simulink model "Project2_Seifi_Ahmadi"  (R2018b)
settings: Solver=ode45  StartTime=0.0  StopTime=900  RelTol=1e-3  EnableMultiTasking=on
values from neighbouring files (symbols this model uses):
  P1 = tf(num,den,'InputDelay',L)    [Project2_Seyfi_Ahmadi.m]
  P2 = tf(num_second,den_second,'InputDelay',190)    [Project2_Seyfi_Ahmadi.m]
undefined symbols (not defined in the file or in its folder): P, tmp
libraries: dspsrcs4 x5
settings Model: TunableVars=tmp  TunableVarsStorageClass=Auto  Creator=Modeer  LastModifiedBy=DearUser
settings DataIOCC: LimitDataPoints=on  SaveFormat=Structure  SaveOutput=off  SaveTime=off
settings OptimizationCC: DefaultParameterBehavior=Inlined  LifeSpan=inf
settings DebuggingCC: UnderspecifiedInitializationDetection=Classic  MergeDetectMultiDrivingBlocksExec=none  SolverPrmCheckMsg=warning  SFUnexpectedBacktrackingDiag=warning  SFNoUnconditionalDefaultTransitionDiag=warning  SFExecutionAtInitializationDiag=none
settings HardwareCC: ProdBitPerPointer=32  ProdBitPerSizeT=32  ProdBitPerPtrDiffT=32  ProdLargestAtomicFloat=None  ProdIntDivRoundTo=Undefined  ProdEndianess=Unspecified  ProdWordSize=32  ProdHWDeviceType=32-bit Generic
settings ModelReferenceCC: PropagateSignalLabelsOutOfModel=off
settings SFSimCC: SimUseLocalCustomCode=off
settings RTWCC: RTWUseLocalCustomCode=off
settings CodeAppCC: StateflowObjectComments=on
settings GRTTargetCC: TargetLangStandard=C89/C90 (ANSI)  GeneratePreprocessorConditionals=Disable all
settings ConfigComp: CovMetricSettings=dw  CovHtmlReporting=on  CovSaveCumulativeToWorkspaceVar=on  CovSaveSingleToWorkspaceVar=on  CovExternalEMLEnable=off

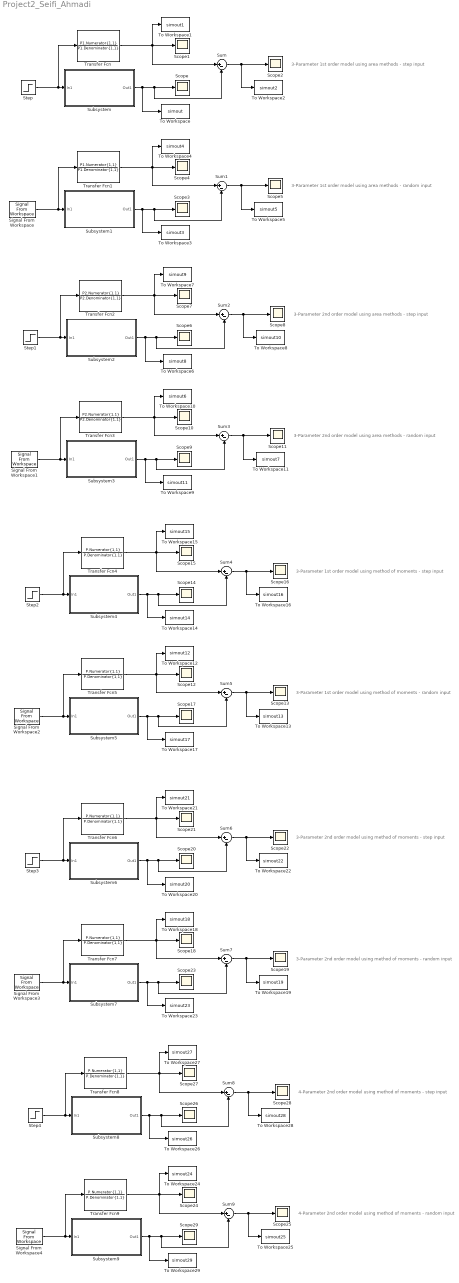
== system Project2_Seifi_Ahmadi ==
  note: 3-Parameter 1st order model using area methods - random input
  note: 3-Parameter 1st order model using area methods - step input
  note: 3-Parameter 2nd order model using area methods - step input
  note: 3-Parameter 2nd order model using area methods - random input
  note: 3-Parameter 1st order model using method of moments - random input
  note: 3-Parameter 1st order model using method of moments - step input
  note: 3-Parameter 2nd order model using method of moments - step input
  note: 3-Parameter 2nd order model using method of moments - random input
  note: 4-Parameter 2nd order model using method of moments - step input
  note: 4-Parameter 2nd order model using method of moments - random input
  Scope{,1..29} (30 alike) : Scope
  Signal From Workspace{,1..4} (5 alike) : dspsrcs4/Signal From Workspace  X=RandomInput  Ts=1  nsamps=1  OutputAfterFinalValue=Setting to zero  ignoreOrWarnInputAndFrameLengths=off  OutputFrames=off
  Step{,1..4} (5 alike) : Step  Time=100  SampleTime=0
  Subsystem : Subsystem  mask{sfcnParam1=tmp}
      mask prompts: sfcnParam1 "tmp:"
      mask help: Simulink:masks:GenSFuncDesc_MD
      mask Help: eval('feval(''rtwprivate'',''rtwhelpview'',''rtw_sfcn_block'')');
  Subsystem1 : Subsystem  mask{sfcnParam1=tmp}
      mask prompts: sfcnParam1 "tmp:"
      mask help: Simulink:masks:GenSFuncDesc_MD
      mask Help: eval('feval(''rtwprivate'',''rtwhelpview'',''rtw_sfcn_block'')');
  Subsystem2 : Subsystem  mask{sfcnParam1=tmp}
      mask prompts: sfcnParam1 "tmp:"
      mask help: Simulink:masks:GenSFuncDesc_MD
      mask Help: eval('feval(''rtwprivate'',''rtwhelpview'',''rtw_sfcn_block'')');
  Subsystem3 : Subsystem  mask{sfcnParam1=tmp}
      mask prompts: sfcnParam1 "tmp:"
      mask help: Simulink:masks:GenSFuncDesc_MD
      mask Help: eval('feval(''rtwprivate'',''rtwhelpview'',''rtw_sfcn_block'')');
  Subsystem4 : Subsystem  mask{sfcnParam1=tmp}
      mask prompts: sfcnParam1 "tmp:"
      mask help: Simulink:masks:GenSFuncDesc_MD
      mask Help: eval('feval(''rtwprivate'',''rtwhelpview'',''rtw_sfcn_block'')');
  Subsystem5 : Subsystem  mask{sfcnParam1=tmp}
      mask prompts: sfcnParam1 "tmp:"
      mask help: Simulink:masks:GenSFuncDesc_MD
      mask Help: eval('feval(''rtwprivate'',''rtwhelpview'',''rtw_sfcn_block'')');
  Subsystem6 : Subsystem  mask{sfcnParam1=tmp}
      mask prompts: sfcnParam1 "tmp:"
      mask help: Simulink:masks:GenSFuncDesc_MD
      mask Help: eval('feval(''rtwprivate'',''rtwhelpview'',''rtw_sfcn_block'')');
  Subsystem7 : Subsystem  mask{sfcnParam1=tmp}
      mask prompts: sfcnParam1 "tmp:"
      mask help: Simulink:masks:GenSFuncDesc_MD
      mask Help: eval('feval(''rtwprivate'',''rtwhelpview'',''rtw_sfcn_block'')');
  Subsystem8 : Subsystem  mask{sfcnParam1=tmp}
      mask prompts: sfcnParam1 "tmp:"
      mask help: Simulink:masks:GenSFuncDesc_MD
      mask Help: eval('feval(''rtwprivate'',''rtwhelpview'',''rtw_sfcn_block'')');
  Subsystem9 : Subsystem  mask{sfcnParam1=tmp}
      mask prompts: sfcnParam1 "tmp:"
      mask help: Simulink:masks:GenSFuncDesc_MD
      mask Help: eval('feval(''rtwprivate'',''rtwhelpview'',''rtw_sfcn_block'')');
  Sum{,1..9} (10 alike) : Sum  Inputs=|+-
  To Workspace : ToWorkspace  VariableName=simout  SaveFormat=Timeseries  SampleTime=-1
  To Workspace1 : ToWorkspace  VariableName=simout1  SaveFormat=Timeseries  SampleTime=-1
  To Workspace10 : ToWorkspace  VariableName=simout6  SaveFormat=Timeseries  SampleTime=-1
  To Workspace11 : ToWorkspace  VariableName=simout7  SaveFormat=Timeseries  SampleTime=-1
  To Workspace12 : ToWorkspace  VariableName=simout12  SaveFormat=Timeseries  SampleTime=-1
  To Workspace13 : ToWorkspace  VariableName=simout13  SaveFormat=Timeseries  SampleTime=-1
  To Workspace14 : ToWorkspace  VariableName=simout14  SaveFormat=Timeseries  SampleTime=-1
  To Workspace15 : ToWorkspace  VariableName=simout15  SaveFormat=Timeseries  SampleTime=-1
  To Workspace16 : ToWorkspace  VariableName=simout16  SaveFormat=Timeseries  SampleTime=-1
  To Workspace17 : ToWorkspace  VariableName=simout17  SaveFormat=Timeseries  SampleTime=-1
  To Workspace18 : ToWorkspace  VariableName=simout18  SaveFormat=Timeseries  SampleTime=-1
  To Workspace19 : ToWorkspace  VariableName=simout19  SaveFormat=Timeseries  SampleTime=-1
  To Workspace2 : ToWorkspace  VariableName=simout2  SaveFormat=Timeseries  SampleTime=-1
  To Workspace20 : ToWorkspace  VariableName=simout20  SaveFormat=Timeseries  SampleTime=-1
  To Workspace21 : ToWorkspace  VariableName=simout21  SaveFormat=Timeseries  SampleTime=-1
  To Workspace22 : ToWorkspace  VariableName=simout22  SaveFormat=Timeseries  SampleTime=-1
  To Workspace23 : ToWorkspace  VariableName=simout23  SaveFormat=Timeseries  SampleTime=-1
  To Workspace24 : ToWorkspace  VariableName=simout24  SaveFormat=Timeseries  SampleTime=-1
  To Workspace25 : ToWorkspace  VariableName=simout25  SaveFormat=Timeseries  SampleTime=-1
  To Workspace26 : ToWorkspace  VariableName=simout26  SaveFormat=Timeseries  SampleTime=-1
  To Workspace27 : ToWorkspace  VariableName=simout27  SaveFormat=Timeseries  SampleTime=-1
  To Workspace28 : ToWorkspace  VariableName=simout28  SaveFormat=Timeseries  SampleTime=-1
  To Workspace29 : ToWorkspace  VariableName=simout29  SaveFormat=Timeseries  SampleTime=-1
  To Workspace3 : ToWorkspace  VariableName=simout3  SaveFormat=Timeseries  SampleTime=-1
  To Workspace4 : ToWorkspace  VariableName=simout4  SaveFormat=Timeseries  SampleTime=-1
  To Workspace5 : ToWorkspace  VariableName=simout5  SaveFormat=Timeseries  SampleTime=-1
  To Workspace6 : ToWorkspace  VariableName=simout8  SaveFormat=Timeseries  SampleTime=-1
  To Workspace7 : ToWorkspace  VariableName=simout9  SaveFormat=Timeseries  SampleTime=-1
  To Workspace8 : ToWorkspace  VariableName=simout10  SaveFormat=Timeseries  SampleTime=-1
  To Workspace9 : ToWorkspace  VariableName=simout11  SaveFormat=Timeseries  SampleTime=-1
  Transfer Fcn : TransferFcn  Numerator=P1.Numerator{1,1}  Denominator=P1.Denominator{1,1}
  Transfer Fcn1 : TransferFcn  Numerator=P1.Numerator{1,1}  Denominator=P1.Denominator{1,1}
  Transfer Fcn2 : TransferFcn  Numerator=P2.Numerator{1,1}  Denominator=P2.Denominator{1,1}
  Transfer Fcn3 : TransferFcn  Numerator=P2.Numerator{1,1}  Denominator=P2.Denominator{1,1}
  Transfer Fcn{4..9} (6 alike) : TransferFcn  Numerator=P.Numerator{1,1}  Denominator=P.Denominator{1,1}
  wires:
  Step/1 -> Transfer Fcn/1, Subsystem/1(In1)
  Subsystem/1(Out1) -> To Workspace/1, Sum/2, Scope/1
  Transfer Fcn/1 -> To Workspace1/1, Scope1/1, Sum/1
  Sum/1 -> To Workspace2/1, Scope2/1
  Subsystem1/1(Out1) -> To Workspace3/1, Sum1/2, Scope3/1
  Signal From Workspace/1 -> Transfer Fcn1/1, Subsystem1/1(In1)
  Transfer Fcn1/1 -> To Workspace4/1, Scope4/1, Sum1/1
  Sum1/1 -> To Workspace5/1, Scope5/1
  Sum3/1 -> To Workspace11/1, Scope11/1
  Transfer Fcn3/1 -> To Workspace10/1, Scope10/1, Sum3/1
  Subsystem2/1(Out1) -> To Workspace6/1, Sum2/2, Scope6/1
  Step1/1 -> Transfer Fcn2/1, Subsystem2/1(In1)
  Transfer Fcn2/1 -> To Workspace7/1, Scope7/1, Sum2/1
  Signal From Workspace1/1 -> Transfer Fcn3/1, Subsystem3/1(In1)
  Subsystem3/1(Out1) -> To Workspace9/1, Sum3/2, Scope9/1
  Sum2/1 -> To Workspace8/1, Scope8/1
  Sum4/1 -> To Workspace16/1, Scope16/1
  Subsystem5/1(Out1) -> To Workspace17/1, Sum5/2, Scope17/1
  Signal From Workspace2/1 -> Transfer Fcn5/1, Subsystem5/1(In1)
  Transfer Fcn4/1 -> To Workspace15/1, Scope15/1, Sum4/1
  Step2/1 -> Transfer Fcn4/1, Subsystem4/1(In1)
  Subsystem4/1(Out1) -> To Workspace14/1, Sum4/2, Scope14/1
  Transfer Fcn5/1 -> To Workspace12/1, Scope12/1, Sum5/1
  Sum5/1 -> To Workspace13/1, Scope13/1
  Subsystem6/1(Out1) -> To Workspace20/1, Sum6/2, Scope20/1
  Transfer Fcn7/1 -> To Workspace18/1, Scope18/1, Sum7/1
  Transfer Fcn6/1 -> To Workspace21/1, Scope21/1, Sum6/1
  Signal From Workspace3/1 -> Transfer Fcn7/1, Subsystem7/1(In1)
  Step3/1 -> Transfer Fcn6/1, Subsystem6/1(In1)
  Sum7/1 -> To Workspace19/1, Scope19/1
  Subsystem7/1(Out1) -> To Workspace23/1, Sum7/2, Scope23/1
  Sum6/1 -> To Workspace22/1, Scope22/1
  Step4/1 -> Transfer Fcn8/1, Subsystem8/1(In1)
  Sum9/1 -> To Workspace25/1, Scope25/1
  Signal From Workspace4/1 -> Transfer Fcn9/1, Subsystem9/1(In1)
  Transfer Fcn8/1 -> To Workspace27/1, Scope27/1, Sum8/1
  Transfer Fcn9/1 -> To Workspace24/1, Scope24/1, Sum9/1
  Sum8/1 -> To Workspace28/1, Scope28/1
  Subsystem8/1(Out1) -> To Workspace26/1, Sum8/2, Scope26/1
  Subsystem9/1(Out1) -> To Workspace29/1, Sum9/2, Scope29/1

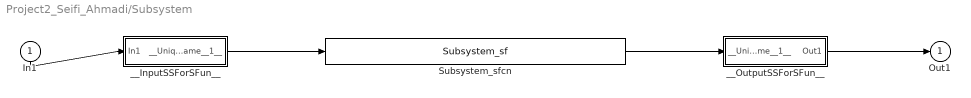
== system Project2_Seifi_Ahmadi/Subsystem ==
  In1 : Inport
  Subsystem_sfcn : S-Function  FunctionName=Subsystem_sf  Parameters=sfcnParam1  SFunctionModules=""  SFunctionDeploymentMode=off  EnableBusSupport=off  mask{rtw_sf_name=Subsystem_sf, showVar=off, sfcnParam1=sfcnParam1}
      mask prompts: rtw_sf_name "Simulink:masks:GenSFuncName_MP"; showVar "Simulink:masks:GenSFuncShowModuleList_MP"; sfcnParam1 "tmp:"
      mask help: Simulink:masks:GenSFuncDesc_MD
      mask init:
      | displist = '';
      | if ~strcmp(get_param(gcb, 'FunctionName'), rtw_sf_name);
      |   set_param(gcb, 'FunctionName', rtw_sf_name);
      | end
      | % Check if we are generating code
      | rtw_mode = false;
      | if strcmpi(get_param(bdroot(gcb),'SimulationStatus'),'Initializing')
      | 	rtw_mode = strcmpi(get_param(bdroot(gcb),'BuildingRTWCode'),'on') && ...
      | 		~strcmpi(get_param(bdroot(gcb),'TargetStyle'),'SimulationTarget');
      | end
      | if showVar || rtw_mode
      | 	if exist('rtwsfunc') == 2 | exist('rtwsfunc') == 6
      | 		tmplist = rtwsfunc(rtw_sf_name,gcb);
      | 		tmplist = DAStudio.message('Simulink:masks:GenSFuncListOfModules_IC', tmplist);
      | 	elseif showVar
      | 		tmplist1 = DAStudio.message('Simulink:masks:GenSFuncListOfModules_IC', '');
      |         tmplist2 = DAStudio.message('Simulink:masks:GenSFuncNotLicensed_IC');
      |         tmplist = [tmplist1 tmplist2];
      |  	end
      | end
      | if showVar
      |   displist = tmplist;
      | end
      settings: CopyFcn=|
      | if ~strcmp(get_param(gcb,'Linkstatus'),'none') && ...
      | ~strcmp(get_param(gcb,'Linkstatus'),'implicit')
      |   set_param(gcb,'LinkStatus','none');
      | end
      mask Help: eval('feval(''rtwprivate'',''rtwhelpview'',''rtw_sfcn_block'')');
      mask Display:
      | port_label('input',1,'In1');
      | port_label('output',1,'Out1');
  __InputSSForSFun__ : Subsystem
  __OutputSSForSFun__ : Subsystem
  Out1 : Outport
  wires:
  In1/1 -> __InputSSForSFun__/1(In1)
  __InputSSForSFun__/1(__UniqueOutportName__1__) -> Subsystem_sfcn/1
  Subsystem_sfcn/1 -> __OutputSSForSFun__/1(__UniqueInportName__1__)
  __OutputSSForSFun__/1(Out1) -> Out1/1

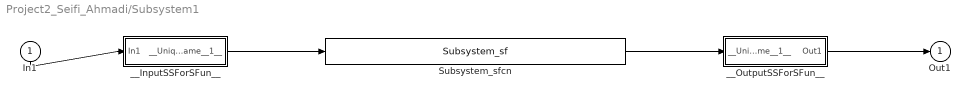
== system Project2_Seifi_Ahmadi/Subsystem1 ==
  In1 : Inport
  Subsystem_sfcn : S-Function  FunctionName=Subsystem_sf  Parameters=sfcnParam1  SFunctionModules=""  SFunctionDeploymentMode=off  EnableBusSupport=off  mask{rtw_sf_name=Subsystem_sf, showVar=off, sfcnParam1=sfcnParam1}
      mask prompts: rtw_sf_name "Simulink:masks:GenSFuncName_MP"; showVar "Simulink:masks:GenSFuncShowModuleList_MP"; sfcnParam1 "tmp:"
      mask help: Simulink:masks:GenSFuncDesc_MD
      mask init: same as Project2_Seifi_Ahmadi/Subsystem/Subsystem_sfcn
      settings: CopyFcn=|
      | if ~strcmp(get_param(gcb,'Linkstatus'),'none') && ...
      | ~strcmp(get_param(gcb,'Linkstatus'),'implicit')
      |   set_param(gcb,'LinkStatus','none');
      | end
      mask Help: eval('feval(''rtwprivate'',''rtwhelpview'',''rtw_sfcn_block'')');
      mask Display:
      | port_label('input',1,'In1');
      | port_label('output',1,'Out1');
  __InputSSForSFun__ : Subsystem
  __OutputSSForSFun__ : Subsystem
  Out1 : Outport
  wires:
  In1/1 -> __InputSSForSFun__/1(In1)
  __InputSSForSFun__/1(__UniqueOutportName__1__) -> Subsystem_sfcn/1
  Subsystem_sfcn/1 -> __OutputSSForSFun__/1(__UniqueInportName__1__)
  __OutputSSForSFun__/1(Out1) -> Out1/1

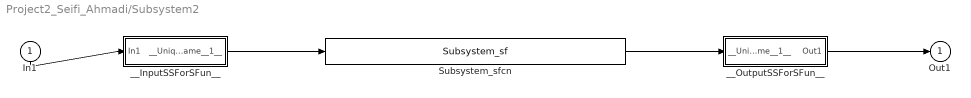
== system Project2_Seifi_Ahmadi/Subsystem2 ==
  In1 : Inport
  Subsystem_sfcn : S-Function  FunctionName=Subsystem_sf  Parameters=sfcnParam1  SFunctionModules=""  SFunctionDeploymentMode=off  EnableBusSupport=off  mask{rtw_sf_name=Subsystem_sf, showVar=off, sfcnParam1=sfcnParam1}
      mask prompts: rtw_sf_name "Simulink:masks:GenSFuncName_MP"; showVar "Simulink:masks:GenSFuncShowModuleList_MP"; sfcnParam1 "tmp:"
      mask help: Simulink:masks:GenSFuncDesc_MD
      mask init: same as Project2_Seifi_Ahmadi/Subsystem/Subsystem_sfcn
      settings: CopyFcn=|
      | if ~strcmp(get_param(gcb,'Linkstatus'),'none') && ...
      | ~strcmp(get_param(gcb,'Linkstatus'),'implicit')
      |   set_param(gcb,'LinkStatus','none');
      | end
      mask Help: eval('feval(''rtwprivate'',''rtwhelpview'',''rtw_sfcn_block'')');
      mask Display:
      | port_label('input',1,'In1');
      | port_label('output',1,'Out1');
  __InputSSForSFun__ : Subsystem
  __OutputSSForSFun__ : Subsystem
  Out1 : Outport
  wires:
  In1/1 -> __InputSSForSFun__/1(In1)
  __InputSSForSFun__/1(__UniqueOutportName__1__) -> Subsystem_sfcn/1
  Subsystem_sfcn/1 -> __OutputSSForSFun__/1(__UniqueInportName__1__)
  __OutputSSForSFun__/1(Out1) -> Out1/1

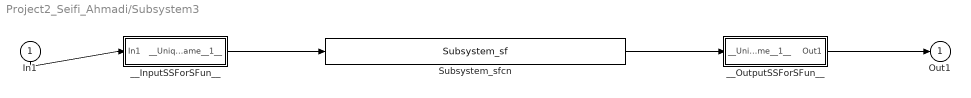
== system Project2_Seifi_Ahmadi/Subsystem3 ==
  In1 : Inport
  Subsystem_sfcn : S-Function  FunctionName=Subsystem_sf  Parameters=sfcnParam1  SFunctionModules=""  SFunctionDeploymentMode=off  EnableBusSupport=off  mask{rtw_sf_name=Subsystem_sf, showVar=off, sfcnParam1=sfcnParam1}
      mask prompts: rtw_sf_name "Simulink:masks:GenSFuncName_MP"; showVar "Simulink:masks:GenSFuncShowModuleList_MP"; sfcnParam1 "tmp:"
      mask help: Simulink:masks:GenSFuncDesc_MD
      mask init: same as Project2_Seifi_Ahmadi/Subsystem/Subsystem_sfcn
      settings: CopyFcn=|
      | if ~strcmp(get_param(gcb,'Linkstatus'),'none') && ...
      | ~strcmp(get_param(gcb,'Linkstatus'),'implicit')
      |   set_param(gcb,'LinkStatus','none');
      | end
      mask Help: eval('feval(''rtwprivate'',''rtwhelpview'',''rtw_sfcn_block'')');
      mask Display:
      | port_label('input',1,'In1');
      | port_label('output',1,'Out1');
  __InputSSForSFun__ : Subsystem
  __OutputSSForSFun__ : Subsystem
  Out1 : Outport
  wires:
  In1/1 -> __InputSSForSFun__/1(In1)
  __InputSSForSFun__/1(__UniqueOutportName__1__) -> Subsystem_sfcn/1
  Subsystem_sfcn/1 -> __OutputSSForSFun__/1(__UniqueInportName__1__)
  __OutputSSForSFun__/1(Out1) -> Out1/1

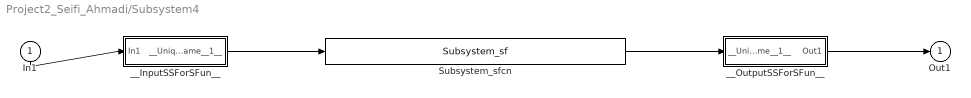
== system Project2_Seifi_Ahmadi/Subsystem4 ==
  In1 : Inport
  Subsystem_sfcn : S-Function  FunctionName=Subsystem_sf  Parameters=sfcnParam1  SFunctionModules=""  SFunctionDeploymentMode=off  EnableBusSupport=off  mask{rtw_sf_name=Subsystem_sf, showVar=off, sfcnParam1=sfcnParam1}
      mask prompts: rtw_sf_name "Simulink:masks:GenSFuncName_MP"; showVar "Simulink:masks:GenSFuncShowModuleList_MP"; sfcnParam1 "tmp:"
      mask help: Simulink:masks:GenSFuncDesc_MD
      mask init: same as Project2_Seifi_Ahmadi/Subsystem/Subsystem_sfcn
      settings: CopyFcn=|
      | if ~strcmp(get_param(gcb,'Linkstatus'),'none') && ...
      | ~strcmp(get_param(gcb,'Linkstatus'),'implicit')
      |   set_param(gcb,'LinkStatus','none');
      | end
      mask Help: eval('feval(''rtwprivate'',''rtwhelpview'',''rtw_sfcn_block'')');
      mask Display:
      | port_label('input',1,'In1');
      | port_label('output',1,'Out1');
  __InputSSForSFun__ : Subsystem
  __OutputSSForSFun__ : Subsystem
  Out1 : Outport
  wires:
  In1/1 -> __InputSSForSFun__/1(In1)
  __InputSSForSFun__/1(__UniqueOutportName__1__) -> Subsystem_sfcn/1
  Subsystem_sfcn/1 -> __OutputSSForSFun__/1(__UniqueInportName__1__)
  __OutputSSForSFun__/1(Out1) -> Out1/1

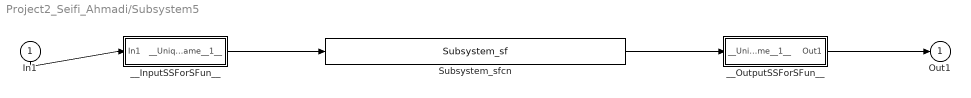
== system Project2_Seifi_Ahmadi/Subsystem5 ==
  In1 : Inport
  Subsystem_sfcn : S-Function  FunctionName=Subsystem_sf  Parameters=sfcnParam1  SFunctionModules=""  SFunctionDeploymentMode=off  EnableBusSupport=off  mask{rtw_sf_name=Subsystem_sf, showVar=off, sfcnParam1=sfcnParam1}
      mask prompts: rtw_sf_name "Simulink:masks:GenSFuncName_MP"; showVar "Simulink:masks:GenSFuncShowModuleList_MP"; sfcnParam1 "tmp:"
      mask help: Simulink:masks:GenSFuncDesc_MD
      mask init: same as Project2_Seifi_Ahmadi/Subsystem/Subsystem_sfcn
      settings: CopyFcn=|
      | if ~strcmp(get_param(gcb,'Linkstatus'),'none') && ...
      | ~strcmp(get_param(gcb,'Linkstatus'),'implicit')
      |   set_param(gcb,'LinkStatus','none');
      | end
      mask Help: eval('feval(''rtwprivate'',''rtwhelpview'',''rtw_sfcn_block'')');
      mask Display:
      | port_label('input',1,'In1');
      | port_label('output',1,'Out1');
  __InputSSForSFun__ : Subsystem
  __OutputSSForSFun__ : Subsystem
  Out1 : Outport
  wires:
  In1/1 -> __InputSSForSFun__/1(In1)
  __InputSSForSFun__/1(__UniqueOutportName__1__) -> Subsystem_sfcn/1
  Subsystem_sfcn/1 -> __OutputSSForSFun__/1(__UniqueInportName__1__)
  __OutputSSForSFun__/1(Out1) -> Out1/1

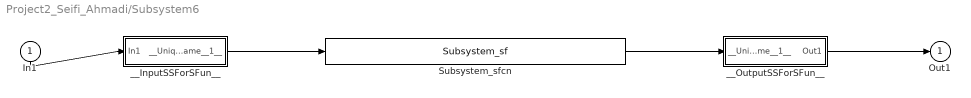
== system Project2_Seifi_Ahmadi/Subsystem6 ==
  In1 : Inport
  Subsystem_sfcn : S-Function  FunctionName=Subsystem_sf  Parameters=sfcnParam1  SFunctionModules=""  SFunctionDeploymentMode=off  EnableBusSupport=off  mask{rtw_sf_name=Subsystem_sf, showVar=off, sfcnParam1=sfcnParam1}
      mask prompts: rtw_sf_name "Simulink:masks:GenSFuncName_MP"; showVar "Simulink:masks:GenSFuncShowModuleList_MP"; sfcnParam1 "tmp:"
      mask help: Simulink:masks:GenSFuncDesc_MD
      mask init: same as Project2_Seifi_Ahmadi/Subsystem/Subsystem_sfcn
      settings: CopyFcn=|
      | if ~strcmp(get_param(gcb,'Linkstatus'),'none') && ...
      | ~strcmp(get_param(gcb,'Linkstatus'),'implicit')
      |   set_param(gcb,'LinkStatus','none');
      | end
      mask Help: eval('feval(''rtwprivate'',''rtwhelpview'',''rtw_sfcn_block'')');
      mask Display:
      | port_label('input',1,'In1');
      | port_label('output',1,'Out1');
  __InputSSForSFun__ : Subsystem
  __OutputSSForSFun__ : Subsystem
  Out1 : Outport
  wires:
  In1/1 -> __InputSSForSFun__/1(In1)
  __InputSSForSFun__/1(__UniqueOutportName__1__) -> Subsystem_sfcn/1
  Subsystem_sfcn/1 -> __OutputSSForSFun__/1(__UniqueInportName__1__)
  __OutputSSForSFun__/1(Out1) -> Out1/1

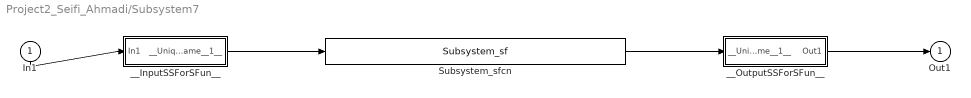
== system Project2_Seifi_Ahmadi/Subsystem7 ==
  In1 : Inport
  Subsystem_sfcn : S-Function  FunctionName=Subsystem_sf  Parameters=sfcnParam1  SFunctionModules=""  SFunctionDeploymentMode=off  EnableBusSupport=off  mask{rtw_sf_name=Subsystem_sf, showVar=off, sfcnParam1=sfcnParam1}
      mask prompts: rtw_sf_name "Simulink:masks:GenSFuncName_MP"; showVar "Simulink:masks:GenSFuncShowModuleList_MP"; sfcnParam1 "tmp:"
      mask help: Simulink:masks:GenSFuncDesc_MD
      mask init: same as Project2_Seifi_Ahmadi/Subsystem/Subsystem_sfcn
      settings: CopyFcn=|
      | if ~strcmp(get_param(gcb,'Linkstatus'),'none') && ...
      | ~strcmp(get_param(gcb,'Linkstatus'),'implicit')
      |   set_param(gcb,'LinkStatus','none');
      | end
      mask Help: eval('feval(''rtwprivate'',''rtwhelpview'',''rtw_sfcn_block'')');
      mask Display:
      | port_label('input',1,'In1');
      | port_label('output',1,'Out1');
  __InputSSForSFun__ : Subsystem
  __OutputSSForSFun__ : Subsystem
  Out1 : Outport
  wires:
  In1/1 -> __InputSSForSFun__/1(In1)
  __InputSSForSFun__/1(__UniqueOutportName__1__) -> Subsystem_sfcn/1
  Subsystem_sfcn/1 -> __OutputSSForSFun__/1(__UniqueInportName__1__)
  __OutputSSForSFun__/1(Out1) -> Out1/1

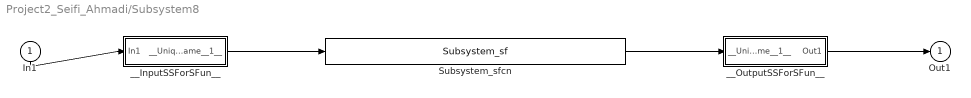
== system Project2_Seifi_Ahmadi/Subsystem8 ==
  In1 : Inport
  Subsystem_sfcn : S-Function  FunctionName=Subsystem_sf  Parameters=sfcnParam1  SFunctionModules=""  SFunctionDeploymentMode=off  EnableBusSupport=off  mask{rtw_sf_name=Subsystem_sf, showVar=off, sfcnParam1=sfcnParam1}
      mask prompts: rtw_sf_name "Simulink:masks:GenSFuncName_MP"; showVar "Simulink:masks:GenSFuncShowModuleList_MP"; sfcnParam1 "tmp:"
      mask help: Simulink:masks:GenSFuncDesc_MD
      mask init: same as Project2_Seifi_Ahmadi/Subsystem/Subsystem_sfcn
      settings: CopyFcn=|
      | if ~strcmp(get_param(gcb,'Linkstatus'),'none') && ...
      | ~strcmp(get_param(gcb,'Linkstatus'),'implicit')
      |   set_param(gcb,'LinkStatus','none');
      | end
      mask Help: eval('feval(''rtwprivate'',''rtwhelpview'',''rtw_sfcn_block'')');
      mask Display:
      | port_label('input',1,'In1');
      | port_label('output',1,'Out1');
  __InputSSForSFun__ : Subsystem
  __OutputSSForSFun__ : Subsystem
  Out1 : Outport
  wires:
  In1/1 -> __InputSSForSFun__/1(In1)
  __InputSSForSFun__/1(__UniqueOutportName__1__) -> Subsystem_sfcn/1
  Subsystem_sfcn/1 -> __OutputSSForSFun__/1(__UniqueInportName__1__)
  __OutputSSForSFun__/1(Out1) -> Out1/1

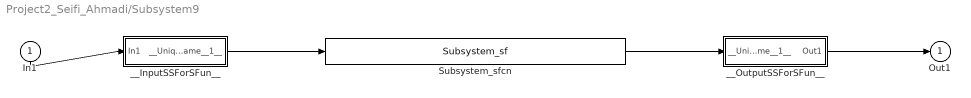
== system Project2_Seifi_Ahmadi/Subsystem9 ==
  In1 : Inport
  Subsystem_sfcn : S-Function  FunctionName=Subsystem_sf  Parameters=sfcnParam1  SFunctionModules=""  SFunctionDeploymentMode=off  EnableBusSupport=off  mask{rtw_sf_name=Subsystem_sf, showVar=off, sfcnParam1=sfcnParam1}
      mask prompts: rtw_sf_name "Simulink:masks:GenSFuncName_MP"; showVar "Simulink:masks:GenSFuncShowModuleList_MP"; sfcnParam1 "tmp:"
      mask help: Simulink:masks:GenSFuncDesc_MD
      mask init: same as Project2_Seifi_Ahmadi/Subsystem/Subsystem_sfcn
      settings: CopyFcn=|
      | if ~strcmp(get_param(gcb,'Linkstatus'),'none') && ...
      | ~strcmp(get_param(gcb,'Linkstatus'),'implicit')
      |   set_param(gcb,'LinkStatus','none');
      | end
      mask Help: eval('feval(''rtwprivate'',''rtwhelpview'',''rtw_sfcn_block'')');
      mask Display:
      | port_label('input',1,'In1');
      | port_label('output',1,'Out1');
  __InputSSForSFun__ : Subsystem
  __OutputSSForSFun__ : Subsystem
  Out1 : Outport
  wires:
  In1/1 -> __InputSSForSFun__/1(In1)
  __InputSSForSFun__/1(__UniqueOutportName__1__) -> Subsystem_sfcn/1
  Subsystem_sfcn/1 -> __OutputSSForSFun__/1(__UniqueInportName__1__)
  __OutputSSForSFun__/1(Out1) -> Out1/1

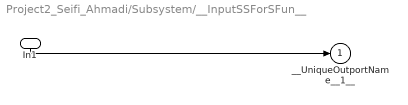
== system Project2_Seifi_Ahmadi/Subsystem/__InputSSForSFun__ ==
  In1 : Inport
  __UniqueOutportName__1__ : Outport
  wires:
  In1/1 -> __UniqueOutportName__1__/1

== system Project2_Seifi_Ahmadi/Subsystem/__OutputSSForSFun__ ==
  __UniqueInportName__1__ : Inport
  Out1 : Outport
  wires:
  __UniqueInportName__1__/1 -> Out1/1

== system Project2_Seifi_Ahmadi/Subsystem1/__InputSSForSFun__ ==
  In1 : Inport
  __UniqueOutportName__1__ : Outport
  wires:
  In1/1 -> __UniqueOutportName__1__/1

== system Project2_Seifi_Ahmadi/Subsystem1/__OutputSSForSFun__ ==
  __UniqueInportName__1__ : Inport
  Out1 : Outport
  wires:
  __UniqueInportName__1__/1 -> Out1/1

== system Project2_Seifi_Ahmadi/Subsystem2/__InputSSForSFun__ ==
  In1 : Inport
  __UniqueOutportName__1__ : Outport
  wires:
  In1/1 -> __UniqueOutportName__1__/1

== system Project2_Seifi_Ahmadi/Subsystem2/__OutputSSForSFun__ ==
  __UniqueInportName__1__ : Inport
  Out1 : Outport
  wires:
  __UniqueInportName__1__/1 -> Out1/1

== system Project2_Seifi_Ahmadi/Subsystem3/__InputSSForSFun__ ==
  In1 : Inport
  __UniqueOutportName__1__ : Outport
  wires:
  In1/1 -> __UniqueOutportName__1__/1

== system Project2_Seifi_Ahmadi/Subsystem3/__OutputSSForSFun__ ==
  __UniqueInportName__1__ : Inport
  Out1 : Outport
  wires:
  __UniqueInportName__1__/1 -> Out1/1

== system Project2_Seifi_Ahmadi/Subsystem4/__InputSSForSFun__ ==
  In1 : Inport
  __UniqueOutportName__1__ : Outport
  wires:
  In1/1 -> __UniqueOutportName__1__/1

== system Project2_Seifi_Ahmadi/Subsystem4/__OutputSSForSFun__ ==
  __UniqueInportName__1__ : Inport
  Out1 : Outport
  wires:
  __UniqueInportName__1__/1 -> Out1/1

== system Project2_Seifi_Ahmadi/Subsystem5/__InputSSForSFun__ ==
  In1 : Inport
  __UniqueOutportName__1__ : Outport
  wires:
  In1/1 -> __UniqueOutportName__1__/1

== system Project2_Seifi_Ahmadi/Subsystem5/__OutputSSForSFun__ ==
  __UniqueInportName__1__ : Inport
  Out1 : Outport
  wires:
  __UniqueInportName__1__/1 -> Out1/1

== system Project2_Seifi_Ahmadi/Subsystem6/__InputSSForSFun__ ==
  In1 : Inport
  __UniqueOutportName__1__ : Outport
  wires:
  In1/1 -> __UniqueOutportName__1__/1

== system Project2_Seifi_Ahmadi/Subsystem6/__OutputSSForSFun__ ==
  __UniqueInportName__1__ : Inport
  Out1 : Outport
  wires:
  __UniqueInportName__1__/1 -> Out1/1

== system Project2_Seifi_Ahmadi/Subsystem7/__InputSSForSFun__ ==
  In1 : Inport
  __UniqueOutportName__1__ : Outport
  wires:
  In1/1 -> __UniqueOutportName__1__/1

== system Project2_Seifi_Ahmadi/Subsystem7/__OutputSSForSFun__ ==
  __UniqueInportName__1__ : Inport
  Out1 : Outport
  wires:
  __UniqueInportName__1__/1 -> Out1/1

== system Project2_Seifi_Ahmadi/Subsystem8/__InputSSForSFun__ ==
  In1 : Inport
  __UniqueOutportName__1__ : Outport
  wires:
  In1/1 -> __UniqueOutportName__1__/1

== system Project2_Seifi_Ahmadi/Subsystem8/__OutputSSForSFun__ ==
  __UniqueInportName__1__ : Inport
  Out1 : Outport
  wires:
  __UniqueInportName__1__/1 -> Out1/1

== system Project2_Seifi_Ahmadi/Subsystem9/__InputSSForSFun__ ==
  In1 : Inport
  __UniqueOutportName__1__ : Outport
  wires:
  In1/1 -> __UniqueOutportName__1__/1

== system Project2_Seifi_Ahmadi/Subsystem9/__OutputSSForSFun__ ==
  __UniqueInportName__1__ : Inport
  Out1 : Outport
  wires:
  __UniqueInportName__1__/1 -> Out1/1
